simulink model "SL_Bsp_0"  (R2020a)
settings: Solver=VariableStepAuto  StartTime=0.0  StopTime=10.0  RelTol=1e-3
settings Model: Creator=Horst  LastModifiedBy=Horst
settings DataIOCC: ReturnWorkspaceOutputs=off

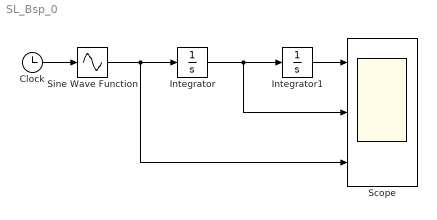
== system SL_Bsp_0 ==
  Clock : Clock
  Integrator : Integrator  InitialCondition=-1
  Integrator1 : Integrator
  Scope : Scope  NumInputPorts=3
  Sine Wave Function : Sin  TimeSource=Use external signal  SampleTime=0
  wires:
  Clock/1 -> Sine Wave Function/1
  Integrator/1 -> Scope/2, Integrator1/1
  Integrator1/1 -> Scope/1
  Sine Wave Function/1 -> Integrator/1, Scope/3
